simulink model "write"  (R2022a)
settings: Solver=FixedStepAuto  StartTime=0.0  StopTime=10.0  RelTol=1e-3  EnableMultiTasking=on
libraries: mbedblockslib x4
settings Model: ExtModeTrigDuration=10  Creator=FUGAZI  LastModifiedBy=FUGAZI
settings OptimizationCC: EnhancedBackFolding=on  PassReuseOutputArgsAs=Individual arguments  ZeroExternalMemoryAtStartup=off  ZeroInternalMemoryAtStartup=off  MaxStackSize=64  OptimizeBlockOrder=speed  DifferentSizesBufferReuse=on  OptimizationCustomize=off  EfficientTunableParamExpr=on
settings DebuggingCC: ParameterTunabilityLossMsg=error  SFUnexpectedBacktrackingDiag=warning  SFNoUnconditionalDefaultTransitionDiag=warning
settings HardwareCC: ProdBitPerPointer=32  ProdBitPerSizeT=32  ProdBitPerPtrDiffT=32  ProdLargestAtomicInteger=Long  ProdLargestAtomicFloat=Double  ProdWordSize=32  ProdLongLongMode=on  ProdHWDeviceType=ARM Compatible->ARM Cortex
settings SFSimCC: MATLABDynamicMemAlloc=off
settings RTWCC: SystemTargetFile=ert.tlc  HardwareBoard=STM32 Nucleo L476RG  TemplateMakefile=ert_default_tmf  GenerateReport=on  Toolchain=GNU Tools for ARM Embedded Processors  BuildConfiguration=Debug  LaunchReport=on
settings CodeAppCC: ForceParamTrailComments=on  IgnoreCustomStorageClasses=off  OperatorAnnotations=on  SimulinkDataObjDesc=on  SFDataObjDesc=on  InsertBlockDesc=on  EnableCustomComments=on
settings ERTTargetCC: ExtModeTransport=3  ExtModeStaticAlloc=on  ExtModeStaticAllocSize=2000  ExtModeMexFile=ext_xcp  ExtModeIntrfLevel=Level2 - Open

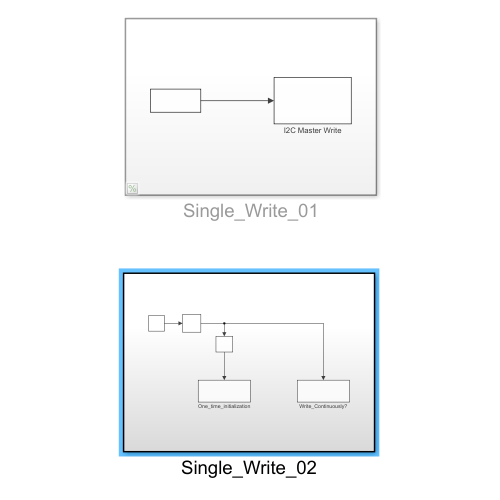
[thumbnail: Simulink's stored preview of the top-level diagram]
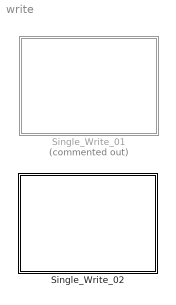
== system write ==
  Single_Write_01 : Subsystem  Commented=on
  Single_Write_02 : Subsystem

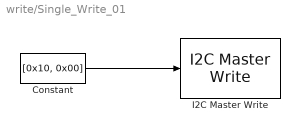
== system write/Single_Write_01 ==
  Constant : Constant  Value=[0x10, 0x00]
  I2C Master Write : mbedblockslib/I2C Master Write  I2CModule=0  Mode=Master  SlaveAddress=hex2dec('40')  SlaveByteOrder=BigEndian  Direction=Transmitter  RegisterAddressMode=on  RegisterAddress=uint8(1)  SlaveDataType=uint8  DataLength=2  NoAck=off  RepeatedStart=off  OutputStatus=off
      settings: SourceProductBaseCode=MICROBIT,NUCLEO,STMICRODIS
  wires:
  Constant/1 -> I2C Master Write/1

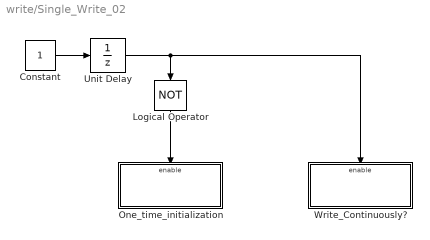
== system write/Single_Write_02 ==
  Constant : Constant  OutDataTypeStr=boolean  SampleTime=0.1
  Logical Operator : Logic  Operator=NOT  AllPortsSameDT=off  OutDataTypeStr=boolean
  One_time_initialization : Subsystem  TreatAsAtomicUnit=on
  Unit Delay : UnitDelay  SampleTime=-1  HasFrameUpgradeWarning=on
  Write_Continuously? : Subsystem  TreatAsAtomicUnit=on
  wires:
  Constant/1 -> Unit Delay/1
  Logical Operator/1 -> One_time_initialization/Enable
  Unit Delay/1 -> Write_Continuously?/Enable, Logical Operator/1

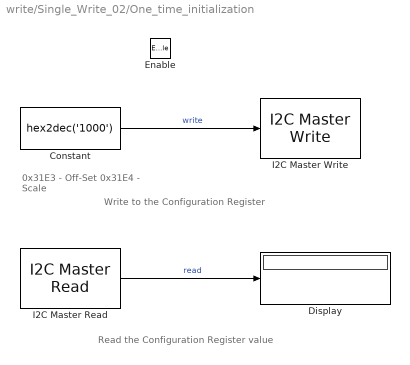
== system write/Single_Write_02/One_time_initialization ==
  note: 0x31E3 - Off-Set
      | 0x31E4 - Scale
  note: Write to the Configuration Register
  note: Read the Configuration Register value
  Enable : EnablePort
  Constant : Constant  Value=hex2dec('1000')  OutDataTypeStr=uint16
  Display : Display
      settings: Format=hex (Stored Integer)
  I2C Master Read : mbedblockslib/I2C Master Read  I2CModule=0  Mode=Master  SlaveAddress=hex2dec('40')  SlaveByteOrder=BigEndian  Direction=Receiver  RegisterAddressMode=on  RegisterAddress=uint8(1)  SlaveDataType=uint16  DataLength=1  NoAck=off  RepeatedStart=off  OutputStatus=off  SampleTime=0.1
      settings: SourceProductBaseCode=MICROBIT,NUCLEO,STMICRODIS
  I2C Master Write : mbedblockslib/I2C Master Write  I2CModule=0  Mode=Master  SlaveAddress=hex2dec('40')  SlaveByteOrder=BigEndian  Direction=Transmitter  RegisterAddressMode=on  RegisterAddress=uint8(1)  SlaveDataType=uint8  DataLength=2  NoAck=off  RepeatedStart=off  OutputStatus=off
      settings: SourceProductBaseCode=MICROBIT,NUCLEO,STMICRODIS
  wires:
  Constant/1 -> I2C Master Write/1  "write"
  I2C Master Read/1 -> Display/1  "read"

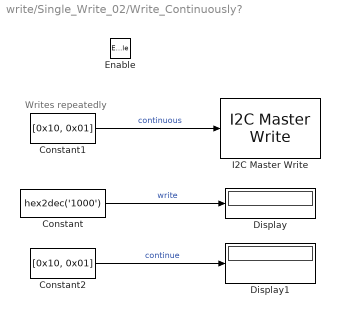
== system write/Single_Write_02/Write_Continuously? ==
  note: Writes repeatedly
  Enable : EnablePort
  Constant : Constant  Value=hex2dec('1000')  OutDataTypeStr=uint16
  Constant1 : Constant  Value=[0x10, 0x01]
  Constant2 : Constant  Value=[0x10, 0x01]
  Display : Display
  Display1 : Display
  I2C Master Write : mbedblockslib/I2C Master Write  I2CModule=0  Mode=Master  SlaveAddress=hex2dec('40')  SlaveByteOrder=BigEndian  Direction=Transmitter  RegisterAddressMode=on  RegisterAddress=uint8(1)  SlaveDataType=uint8  DataLength=2  NoAck=off  RepeatedStart=off  OutputStatus=off
      settings: SourceProductBaseCode=MICROBIT,NUCLEO,STMICRODIS
  wires:
  Constant1/1 -> I2C Master Write/1  "continuous"
  Constant2/1 -> Display1/1  "continue"
  Constant/1 -> Display/1  "write"
